simulink model "SIMULATION_MODEL_v2"  (R2024b)
settings: Solver=VariableStepAuto  StartTime=0.0  StopTime=10.0  RelTol=1e-3
values from neighbouring files (symbols this model uses):
  R = R_roll*R_pitch*R_yaw    [drawCubeSat.m]
undefined symbols (not defined in the file or in its folder): A, Js, juliandate, sat, ws0
libraries: matrix_library x4, aerolibutil x4, sharedtransform x2, sharedutil x1, simulink_extras x1
settings Model: Creator=Ameya  LastModifiedBy=Ameya

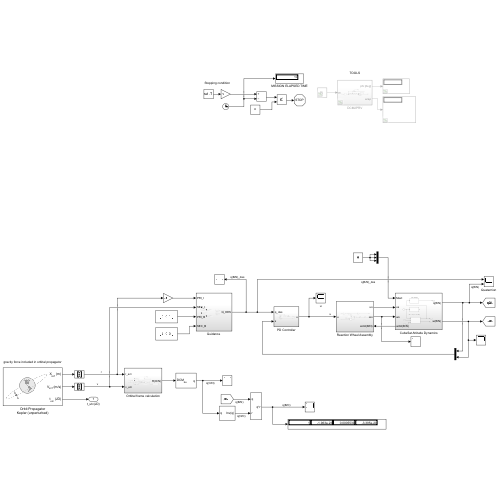
[thumbnail: Simulink's stored preview of the top-level diagram]
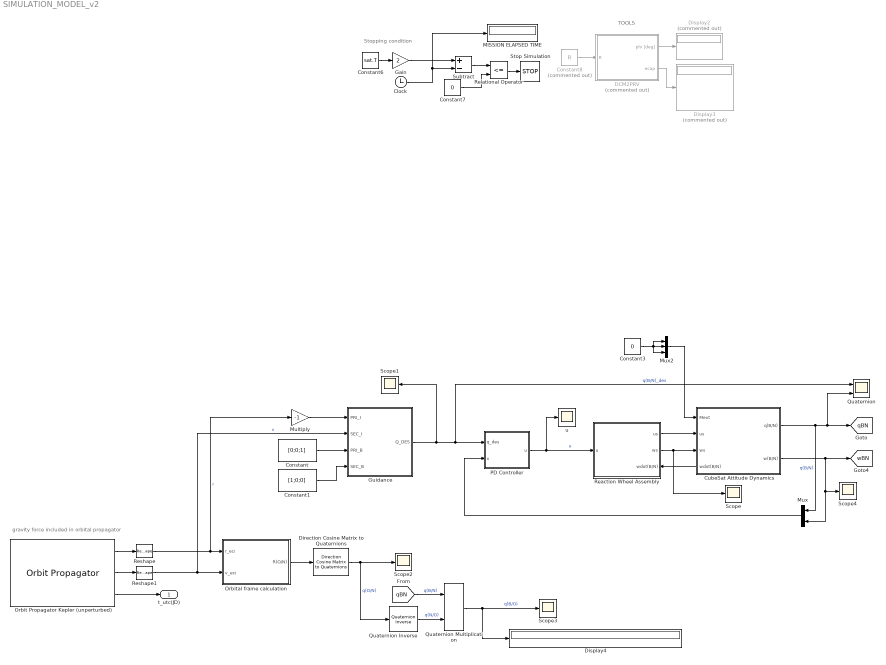
== system SIMULATION_MODEL_v2 ==
  note: TOOLS
  note: Stopping condition
  note: gravity force included in orbital propagator
  Clock : Clock
  Constant : Constant  Value=[0;0;1]  SampleTime=-1
  Constant1 : Constant  Value=[1;0;0]  SampleTime=-1
  Constant3 : Constant  Value=0
  Constant6 : Constant  Value=sat.T
  Constant7 : Constant  Value=0
  Constant8 : Constant  Commented=on  Value=R
  CubeSat Attitude Dynamics : Subsystem
      settings: PortSchema="{\"entries\":[{\"content\":{\"sides\":[{\"content\":{\"connectorIds\":[\"In1\",\"In2\",\"In3\",\"Out3\"]},\"type\":\"ConnectorPlacement.EquallySpacedRectSide\",\"uuid\":\"8820a632-6c9c-47e7-8ef5-be6de2db70d7\"},{\"content\":{\"connectorIds\":[\"Out1\",\"Out2\"],\"side\":\"RIGHT\"},\"type\":\"ConnectorPlacement.EquallySpacedRectSide\",\"uuid\":\"7f0e754f-3cbf-45b6-a264-ccdd31aad370\"},{\"content\":{\"side\":\"TOP\"},\"type\":\"ConnectorPlacement.EquallySpacedRectSide\",\"uuid\":\"2979d5a0-a088-4ee3-9165-a7a9b39adb5e\"}]},\"type\":\"ConnectorPlacement.EquallySpacedConnector\",\"uuid\":\"228422aa-74d2-446a-acdb-f3c611e4b5a7\"}],\"packageUris\":[\"http://schema.mathworks.com/mf0/Connector/R2020b\"],\"version\":\"1.0\"}"
  DCM2PRV : Subsystem  Commented=on
  Direction Cosine Matrix to Quaternions : sharedtransform/Direction Cosine Matrix  to Quaternions  aMode=0  action=Error  tolerance=eps(2)
      settings: LibrarySourceBlock=|
      | aerolibtransform2/Direction Cosine Matrix
      | to Quaternions
  Display2 : Display  Commented=on
  Display3 : Display  Commented=on
  Display4 : Display
  Gain : Gain  Gain=2
  "Guidance " : Subsystem
  MISSION ELAPSED TIME : Display
  Multiply : Gain  Gain=-1
  Mux : Mux  Inputs=2
  Mux2 : Mux  Inputs=3
  Orbit Propagator Kepler (unperturbed) : OrbitPropagator  accelIn=on  startDate=juliandate(2025, 1, 1, 6, 0, 0)  semiMajorAxis=sat.a  eccentricity=sat.e  inclination=rad2deg(sat.i)  raan=rad2deg(sat.RAAN)  argPeriapsis=rad2deg(sat.w)  trueAnomaly=rad2deg(sat.ta)  inertialPosition=[3649700.0 3308200.0 -4676600.0]  inertialVelocity=[-2750.8 6666.4 2573.4]  fixedPosition=[-4142689.0 -2676864.7 -4669861.6]  fixedVelocity=[1452.7 -6720.7 2568.1]  gravityModel=Oblate ellipsoid (J2)  customR=3396200  customMu=4.305e13  customJ2=1.0826269e-03  customOmega=4.06125949e-3
  Orbital frame calculation : Subsystem
  PD Controller : Subsystem
  Quaternion : Scope  NumInputPorts=2
  Quaternion Inverse : aerolibutil/Quaternion Inverse
  Quaternion Multiplication : aerolibutil/Quaternion Multiplication
  Reaction Wheel Assembly : Subsystem
      settings: PortSchema="{\"entries\":[{\"content\":{\"sides\":[{\"content\":{\"connectorIds\":[\"In1\"]},\"type\":\"ConnectorPlacement.EquallySpacedRectSide\",\"uuid\":\"57a5e211-d888-47e5-a410-d74309a415f6\"},{\"content\":{\"connectorIds\":[\"Out1\",\"Out2\",\"In2\"],\"side\":\"RIGHT\"},\"type\":\"ConnectorPlacement.EquallySpacedRectSide\",\"uuid\":\"0d6436a4-96ad-4035-90dd-04c735a462cf\"},{\"content\":{\"side\":\"TOP\"},\"type\":\"ConnectorPlacement.EquallySpacedRectSide\",\"uuid\":\"eefef678-a1c2-433e-9ac3-082bc8edd153\"}]},\"type\":\"ConnectorPlacement.EquallySpacedConnector\",\"uuid\":\"6794547d-8daf-40ab-9bc3-64f70f726c2c\"}],\"packageUris\":[\"http://schema.mathworks.com/mf0/Connector/R2020b\"],\"version\":\"1.0\"}"
  Relational Operator : RelationalOperator  Operator=<=  OutDataTypeStr=boolean  RndMeth=Simplest  InputSameDT=off
  Reshape : Reshape  OutputDimensionality=Column vector (2-D)
  Reshape1 : Reshape  OutputDimensionality=Column vector (2-D)
  Scope{,1..4} (5 alike) : Scope
  Stop Simulation : Stop
  Subtract : Sum  Inputs=+-
  u : Scope
  t_utc(JD) : Outport
  tag scope: qBN=global, wBN=global
  wires:
  Constant/1 -> "Guidance "/3(PRI_B)
  DCM2PRV/2(ecap) -> Display3/1
  Clock/1 -> MISSION ELAPSED TIME/1, Subtract/2
  Orbital frame calculation/1(R(O/N)) -> Direction Cosine Matrix to Quaternions/1
  CubeSat Attitude Dynamics/1(q(B/N)) -> Mux/1, [qBN], Quaternion/2  "q(B/N)"
  CubeSat Attitude Dynamics/2(w(B/N)) -> Mux/2, Scope4/1, [wBN]
  PD Controller/1(u) -> Reaction Wheel Assembly/1(u), u/1  "u"
  Mux/1 -> PD Controller/2(x)
  Relational Operator/1 -> Stop Simulation/1
  Constant3/1 -> Mux2/1, Mux2/3, Mux2/2
  Mux2/1 -> CubeSat Attitude Dynamics/1(Mext)
  Subtract/1 -> Relational Operator/1
  "Guidance "/1(Q_DES) -> Quaternion/1, PD Controller/1(q_des), Scope1/1  "q(B/N)_des"
  Reshape1/1 -> Orbital frame calculation/2(v_eci), "Guidance "/2(SEC_I)  "v"
  Orbit Propagator Kepler (unperturbed)/2 -> Reshape1/1
  Gain/1 -> Subtract/1
  Orbit Propagator Kepler (unperturbed)/1 -> Reshape/1
  Quaternion Inverse/1 -> Quaternion Multiplication/2  "q(N/O)"
  [qBN] -> Quaternion Multiplication/1  "q(B/N)"
  Constant7/1 -> Relational Operator/2
  Constant1/1 -> "Guidance "/4(SEC_B)
  Multiply/1 -> "Guidance "/1(PRI_I)
  Constant6/1 -> Gain/1
  DCM2PRV/1(phi [deg]) -> Display2/1
  Quaternion Multiplication/1 -> Display4/1, Scope3/1  "q(B/O)"
  Reshape/1 -> Multiply/1, Orbital frame calculation/1(r_eci)  "r"
  Constant8/1 -> DCM2PRV/1(R)
  Direction Cosine Matrix to Quaternions/1 -> Scope2/1, Quaternion Inverse/1  "q(O/N)"
  Orbit Propagator Kepler (unperturbed)/3 -> t_utc(JD)/1
  Reaction Wheel Assembly/2(ws) -> Scope/1, CubeSat Attitude Dynamics/3(ws)
  CubeSat Attitude Dynamics/3(wdot(B/N)) -> Reaction Wheel Assembly/2(wdot(B/N))
  Reaction Wheel Assembly/1(us) -> CubeSat Attitude Dynamics/2(us)

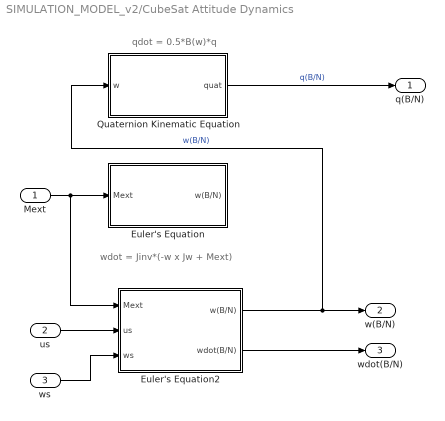
== system SIMULATION_MODEL_v2/CubeSat Attitude Dynamics ==
  note: qdot = 0.5*B(w)*q
  note: wdot = Jinv*(-w x Jw + Mext)
  Mext : Inport
  us : Inport  Port=2
  ws : Inport  Port=3
  Euler's Equation : Subsystem
  Euler's Equation2 : Subsystem
  Quaternion Kinematic Equation : Subsystem
  q(B/N) : Outport
  w(B/N) : Outport  Port=2
  wdot(B/N) : Outport  Port=3
  wires:
  Mext/1 -> Euler's Equation2/1(Mext), Euler's Equation/1(Mext)
  Quaternion Kinematic Equation/1(quat) -> q(B/N)/1  "q(B/N)"
  Euler's Equation2/2(wdot(B/N)) -> wdot(B/N)/1
  us/1 -> Euler's Equation2/2(us)
  ws/1 -> Euler's Equation2/3(ws)
  Euler's Equation2/1(w(B/N)) -> Quaternion Kinematic Equation/1(w), w(B/N)/1  "w(B/N)"

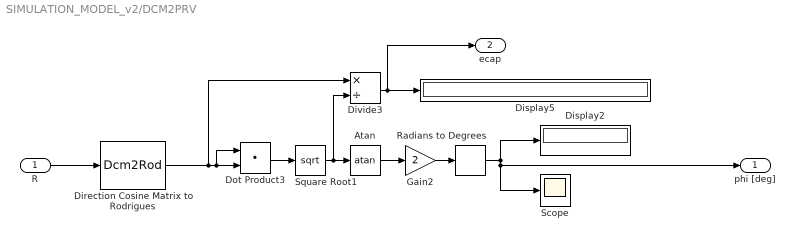
== system SIMULATION_MODEL_v2/DCM2PRV ==
  R : Inport
  Atan : Trigonometry  Operator=atan
  Direction Cosine Matrix to Rodrigues : Dcm2Rod
  Display2 : Display
  Display5 : Display
  Divide3 : Product  Inputs=*/
  Dot Product3 : DotProduct  OutDataTypeStr=Inherit: Inherit via internal rule
  Gain2 : Gain  Gain=2
  Radians to Degrees : simulink_extras/Transformations/Radians to Degrees
  Scope : Scope
  Square Root1 : Sqrt
  phi [deg] : Outport
  ecap : Outport  Port=2
  wires:
  Radians to Degrees/1 -> phi [deg]/1, Scope/1, Display2/1
  Divide3/1 -> ecap/1, Display5/1
  R/1 -> Direction Cosine Matrix to Rodrigues/1
  Square Root1/1 -> Divide3/2, Atan/1
  Atan/1 -> Gain2/1
  Direction Cosine Matrix to Rodrigues/1 -> Divide3/1, Dot Product3/2, Dot Product3/1
  Dot Product3/1 -> Square Root1/1
  Gain2/1 -> Radians to Degrees/1

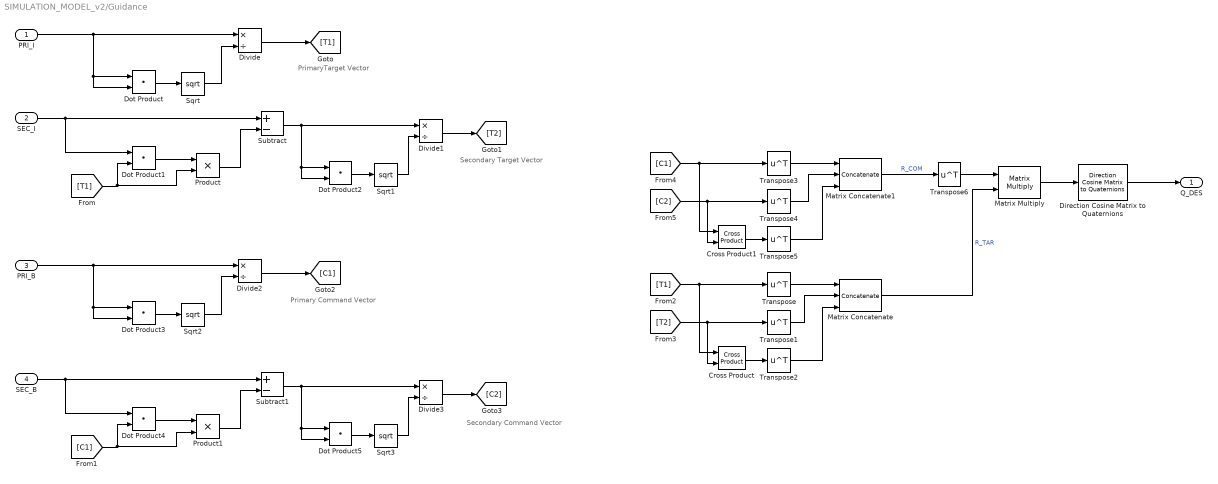
== system SIMULATION_MODEL_v2/Guidance  ==
  note: PrimaryTarget Vector
  note: Secondary Target Vector
  note: Primary Command Vector
  note: Secondary Command Vector
  PRI_I : Inport
  SEC_I : Inport  Port=2
  PRI_B : Inport  Port=3
  SEC_B : Inport  Port=4
  Cross Product : matrix_library/Cross Product
  Cross Product1 : matrix_library/Cross Product
  Direction Cosine Matrix to Quaternions : sharedtransform/Direction Cosine Matrix  to Quaternions  aMode=0  action=None  tolerance=eps(2)
      settings: LibrarySourceBlock=|
      | aerolibtransform2/Direction Cosine Matrix
      | to Quaternions
  Divide{,1..3} (4 alike) : Product  Inputs=*/
  Dot Product{,1..5} (6 alike) : DotProduct  OutDataTypeStr=Inherit: Inherit via internal rule
  Matrix Concatenate : Concatenate  NumInputs=3  Mode=Multidimensional array
  Matrix Concatenate1 : Concatenate  NumInputs=3  Mode=Multidimensional array
  Matrix Multiply : Product  Multiplication=Matrix(*)
  Product : Product
  Product1 : Product
  Sqrt{,1..3} (4 alike) : Sqrt
  Subtract : Sum  Inputs=+-
  Subtract1 : Sum  Inputs=+-
  Transpose{,1..6} (7 alike) : Math  Operator=transpose
  Q_DES : Outport
  wires:
  PRI_I/1 -> Dot Product/2, Dot Product/1, Divide/1
  Dot Product/1 -> Sqrt/1
  Divide/1 -> [T1]
  Transpose/1 -> Matrix Concatenate/1
  SEC_I/1 -> Subtract/1, Dot Product1/1
  Sqrt/1 -> Divide/2
  Dot Product1/1 -> Product/1
  [T1] -> Product/2, Dot Product1/2
  Product/1 -> Subtract/2
  Sqrt1/1 -> Divide1/2
  Dot Product2/1 -> Sqrt1/1
  Subtract/1 -> Divide1/1, Dot Product2/2, Dot Product2/1
  Divide1/1 -> [T2]
  Sqrt2/1 -> Divide2/2
  Dot Product3/1 -> Sqrt2/1
  PRI_B/1 -> Dot Product3/2, Dot Product3/1, Divide2/1
  Divide2/1 -> [C1]
  Dot Product5/1 -> Sqrt3/1
  Sqrt3/1 -> Divide3/2
  Product1/1 -> Subtract1/2
  Divide3/1 -> [C2]
  [C1] -> Product1/2, Dot Product4/2
  Subtract1/1 -> Divide3/1, Dot Product5/2, Dot Product5/1
  Dot Product4/1 -> Product1/1
  SEC_B/1 -> Subtract1/1, Dot Product4/1
  Transpose1/1 -> Matrix Concatenate/2
  Transpose2/1 -> Matrix Concatenate/3
  [T1] -> Cross Product/1, Transpose/1
  [T2] -> Cross Product/2, Transpose1/1
  Cross Product/1 -> Transpose2/1
  Matrix Concatenate/1 -> Matrix Multiply/2  "R_TAR"
  Cross Product1/1 -> Transpose5/1
  [C1] -> Cross Product1/1, Transpose3/1
  Transpose3/1 -> Matrix Concatenate1/1
  Transpose4/1 -> Matrix Concatenate1/2
  Transpose5/1 -> Matrix Concatenate1/3
  [C2] -> Cross Product1/2, Transpose4/1
  Matrix Concatenate1/1 -> Transpose6/1  "R_COM"
  Transpose6/1 -> Matrix Multiply/1
  Matrix Multiply/1 -> Direction Cosine Matrix to Quaternions/1
  Direction Cosine Matrix to Quaternions/1 -> Q_DES/1

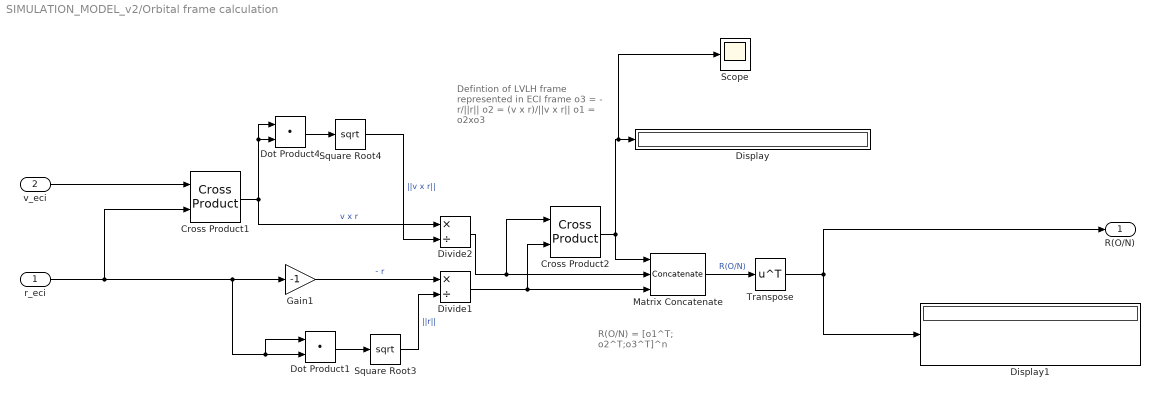
== system SIMULATION_MODEL_v2/Orbital frame calculation ==
  note: R(O/N) = [o1^T; o2^T;o3^T]^n
  note: Defintion of LVLH frame
      | represented in ECI frame
      | o3 = - r/||r||
      | o2 = (v x r)/||v x r||
      | o1 = o2xo3
  r_eci : Inport
  v_eci : Inport  Port=2
  Cross Product1 : matrix_library/Cross Product
  Cross Product2 : matrix_library/Cross Product
  Display : Display
  Display1 : Display
  Divide1 : Product  Inputs=*/
  Divide2 : Product  Inputs=*/
  Dot Product1 : DotProduct  OutDataTypeStr=Inherit: Inherit via internal rule
  Dot Product4 : DotProduct  OutDataTypeStr=Inherit: Inherit via internal rule
  Gain1 : Gain  Gain=-1
  Matrix Concatenate : Concatenate  NumInputs=3  Mode=Multidimensional array  ConcatenateDimension=2
  Scope : Scope
  Square Root3 : Sqrt
  Square Root4 : Sqrt
  Transpose : Math  Operator=transpose
  R(O/N) : Outport
  wires:
  Cross Product2/1 -> Scope/1, Display/1, Matrix Concatenate/1
  Divide2/1 -> Cross Product2/1, Matrix Concatenate/2
  Cross Product1/1 -> Dot Product4/2, Dot Product4/1, Divide2/1  "v x r"
  r_eci/1 -> Cross Product1/2, Dot Product1/1, Dot Product1/2, Gain1/1
  Gain1/1 -> Divide1/1  "- r"
  Square Root3/1 -> Divide1/2  "||r||"
  Square Root4/1 -> Divide2/2  "||v x r||"
  Dot Product1/1 -> Square Root3/1
  v_eci/1 -> Cross Product1/1
  Matrix Concatenate/1 -> Transpose/1  "R(O/N)"
  Divide1/1 -> Cross Product2/2, Matrix Concatenate/3
  Dot Product4/1 -> Square Root4/1
  Transpose/1 -> Display1/1, R(O/N)/1

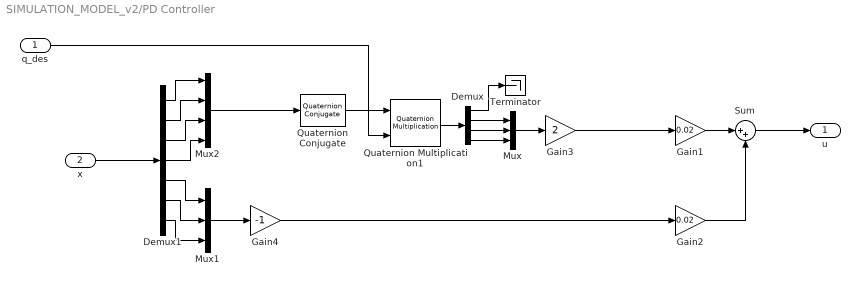
== system SIMULATION_MODEL_v2/PD Controller ==
  q_des : Inport
  x : Inport  Port=2
  Demux : Demux
  Demux1 : Demux  Outputs=7
  Gain1 : Gain  Gain=0.02
  Gain2 : Gain  Gain=0.02
  Gain3 : Gain  Gain=2
  Gain4 : Gain  Gain=-1
  Mux : Mux  Inputs=3
  Mux1 : Mux  Inputs=3
  Mux2 : Mux
  Quaternion Conjugate : aerolibutil/Quaternion Conjugate
  Quaternion Multiplication1 : aerolibutil/Quaternion Multiplication
  Sum : Sum  Inputs=|++
  Terminator : Terminator
  u : Outport
  wires:
  Demux/2 -> Mux/1
  Demux/4 -> Mux/3
  Gain3/1 -> Gain1/1
  Demux/3 -> Mux/2
  Gain2/1 -> Sum/2
  Quaternion Multiplication1/1 -> Demux/1
  Gain4/1 -> Gain2/1
  x/1 -> Demux1/1
  Quaternion Conjugate/1 -> Quaternion Multiplication1/1
  Gain1/1 -> Sum/1
  Mux/1 -> Gain3/1
  Demux/1 -> Terminator/1
  Sum/1 -> u/1
  q_des/1 -> Quaternion Multiplication1/2
  Demux1/5 -> Mux1/1
  Demux1/6 -> Mux1/2
  Demux1/7 -> Mux1/3
  Mux1/1 -> Gain4/1
  Demux1/4 -> Mux2/4
  Demux1/1 -> Mux2/1
  Demux1/2 -> Mux2/2
  Demux1/3 -> Mux2/3
  Mux2/1 -> Quaternion Conjugate/1

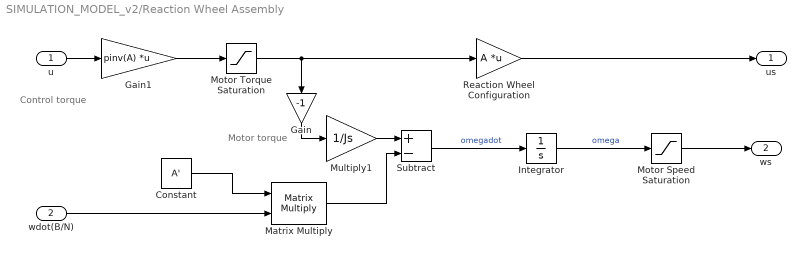
== system SIMULATION_MODEL_v2/Reaction Wheel Assembly ==
  note: Control torque
  note: Motor torque
  u : Inport
  wdot(B/N) : Inport  Port=2
  Constant : Constant  Value=A'
  Gain : Gain  Gain=-1
  Gain1 : Gain  Gain=pinv(A)  Multiplication=Matrix(K*u)
  Integrator : Integrator  InitialCondition=ws0
  Matrix Multiply : Product  Multiplication=Matrix(*)
  Motor Speed Saturation : Saturate  UpperLimit=5000*2*pi/60  LowerLimit=-5000*2*pi/60
  Motor Torque Saturation : Saturate  UpperLimit=0.05  LowerLimit=-0.05
  Multiply1 : Gain  Gain=1/Js
  Reaction Wheel Configuration : Gain  Gain=A  Multiplication=Matrix(K*u)
  Subtract : Sum  Inputs=+-
  us : Outport
  ws : Outport  Port=2
  wires:
  Subtract/1 -> Integrator/1  "omegadot"
  Integrator/1 -> Motor Speed Saturation/1  "omega"
  Motor Torque Saturation/1 -> Reaction Wheel Configuration/1, Gain/1
  u/1 -> Gain1/1
  Multiply1/1 -> Subtract/1
  Matrix Multiply/1 -> Subtract/2
  Motor Speed Saturation/1 -> ws/1
  Gain/1 -> Multiply1/1
  Gain1/1 -> Motor Torque Saturation/1
  Reaction Wheel Configuration/1 -> us/1
  Constant/1 -> Matrix Multiply/1
  wdot(B/N)/1 -> Matrix Multiply/2

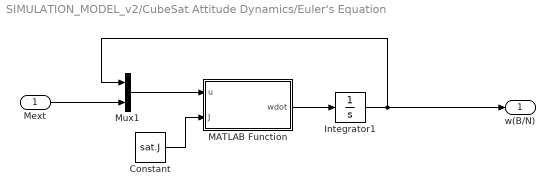
== system SIMULATION_MODEL_v2/CubeSat Attitude Dynamics/Euler's Equation ==
  Mext : Inport
  Constant : Constant  Value=sat.J
  Integrator1 : Integrator  InitialCondition=sat.omegaBO
  MATLAB Function : MATLAB Function  TreatAsAtomicUnit=on
  Mux1 : Mux  Inputs=2
  w(B/N) : Outport
  wires:
  Mext/1 -> Mux1/2
  MATLAB Function/1(wdot) -> Integrator1/1
  Integrator1/1 -> Mux1/1, w(B/N)/1
  Mux1/1 -> MATLAB Function/1(u)
  Constant/1 -> MATLAB Function/2(J)

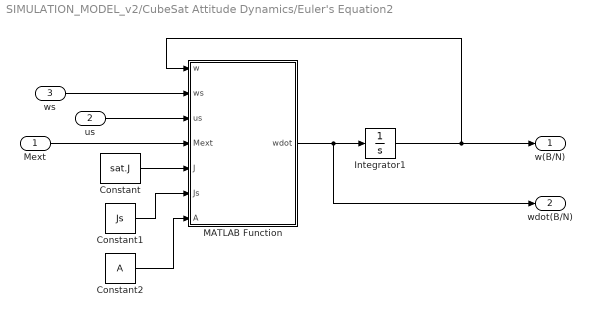
== system SIMULATION_MODEL_v2/CubeSat Attitude Dynamics/Euler's Equation2 ==
  Mext : Inport
  us : Inport  Port=2
  ws : Inport  Port=3
  Constant : Constant  Value=sat.J
  Constant1 : Constant  Value=Js
  Constant2 : Constant  Value=A
  Integrator1 : Integrator  InitialCondition=sat.omegaBN
  MATLAB Function : MATLAB Function  TreatAsAtomicUnit=on
  w(B/N) : Outport
  wdot(B/N) : Outport  Port=2
  wires:
  MATLAB Function/1(wdot) -> wdot(B/N)/1, Integrator1/1
  Integrator1/1 -> MATLAB Function/1(w), w(B/N)/1
  ws/1 -> MATLAB Function/2(ws)
  Constant/1 -> MATLAB Function/5(J)
  Constant1/1 -> MATLAB Function/6(Js)
  Constant2/1 -> MATLAB Function/7(A)
  Mext/1 -> MATLAB Function/4(Mext)
  us/1 -> MATLAB Function/3(us)

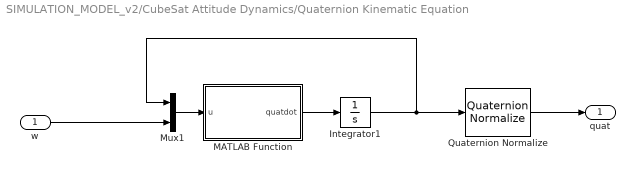
== system SIMULATION_MODEL_v2/CubeSat Attitude Dynamics/Quaternion Kinematic Equation ==
  w : Inport
  Integrator1 : Integrator  InitialCondition=sat.quat
  MATLAB Function : MATLAB Function  TreatAsAtomicUnit=on
  Mux1 : Mux  Inputs=2
  Quaternion Normalize : sharedutil/Quaternion Normalize  aMode=aMode
  quat : Outport
  wires:
  Mux1/1 -> MATLAB Function/1(u)
  Integrator1/1 -> Quaternion Normalize/1, Mux1/1
  MATLAB Function/1(quatdot) -> Integrator1/1
  w/1 -> Mux1/2
  Quaternion Normalize/1 -> quat/1

== matlab function SIMULATION_MODEL_v2/CubeSat Attitude Dynamics/Quaternion Kinematic Equation/MATLAB Function ==
  data: u input; quatdot output
function quatdot = quatKinematics(u)
    quat = u(1:4);
    p = u(5);
    q = u(6);
    r = u(7);
    quatdot = 0.5*[0,-p,-q,-r;
                p,0,r,-q;
                q,-r,0,p;
                r,q,-p,0]*quat;
end

== matlab function SIMULATION_MODEL_v2/CubeSat Attitude Dynamics/Euler's Equation/MATLAB Function ==
  data: u input; wdot output; J input
function wdot = EulersEOM(u,J)
    w = u(1:3);
    m = u(4:6);
    wdot = J\(-cross(w,(J*w))+m);
end

== matlab function SIMULATION_MODEL_v2/CubeSat Attitude Dynamics/Euler's Equation2/MATLAB Function ==
  data: w input; ws input; us input; Mext input; wdot output; J input; Js input; A input
function wdot = EulersEOM(w,ws,us,Mext,J,Js,A)
    Jbar = J - (A*Js*A');
    hs = Js*(ws+A'*w);
    wdot = Jbar\(Mext+ us -cross(w,(Jbar*w + A*hs)));
end
